simulink model "sampleModel1989"  (R2023a)
settings: Solver=VariableStepAuto  StartTime=0.0  StopTime=10.0  RelTol=1e-3
libraries: hdlsllib x7, simulink x2
settings Model: Creator=user1  LastModifiedBy=user1

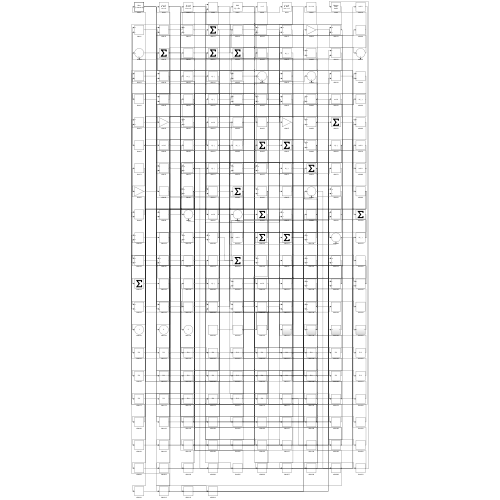
[thumbnail: Simulink's stored preview of the top-level diagram]
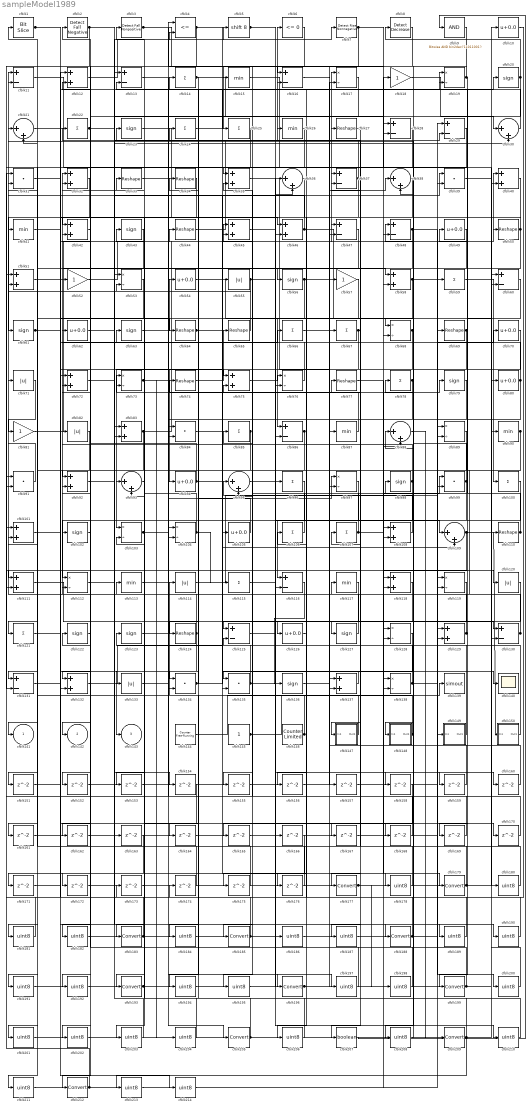
== system sampleModel1989 ==
  cfblk1 : hdlsllib/Logic and Bit Operations/Bit Slice  lidx=7  ridx=0
  cfblk{10,49,54,62,70,80,94,105,126} (9 alike) : Bias  Bias=0.0  SaturateOnIntegerOverflow=off
  cfblk{14,22,24..25,59,66..67,78,85,96,100,106..107,115,121} (15 alike) : Sum  Inputs=+
  cfblk{12,32,35,40,42,45..46,51,58,72,75,83,92,101,108,111,118,129,132,137} (20 alike) : Sum
  cfblk{20,23,43,56,61,63,79,98,102,122..123,127,136} (13 alike) : Signum
  cfblk{17,19,53,68,73,76,89,97,103..104,112,119,128,138} (14 alike) : Product  Inputs=*/  RndMeth=Zero  SaturateOnIntegerOverflow=on
  cfblk{21,30,36,38,88,93,95,109} (8 alike) : Sum  Inputs=|++
  cfblk{11,13,16,28..29,37,47..48,60,86,116,125,130..131} (14 alike) : Sum  Inputs=+-
  cfblk{27,33..34,44,50,64..65,69,74,77,110,124} (12 alike) : Reshape
  cfblk{15,26,41,87,90,113,117} (7 alike) : MinMax
  cfblk{55,71,82,114,120,133} (6 alike) : Abs  SaturateOnIntegerOverflow=off
  cfblk{31,39,84,91,99,134..135} (7 alike) : DotProduct  OutDataTypeStr=Inherit: Inherit via internal rule
  cfblk139 : ToWorkspace  VariableName=simout  SaveFormat=Timeseries  SampleTime=-1
  cfblk140 : Scope
  cfblk144 : hdlsllib/Sources/Counter Free-Running  NumBits=16  tsamp=-1
  cfblk145 : Constant  SampleTime=-1
  cfblk146 : hdlsllib/Sources/Counter Limited  uplimit=7  tsamp=-1
  cfblk147 : Subsystem
      settings: LibrarySourceBlock=|
      | hdlsllib/Ports &
      | Subsystems/Subsystem
  cfblk148 : Subsystem
      settings: LibrarySourceBlock=|
      | hdlsllib/Ports &
      | Subsystems/Subsystem
  cfblk149 : Subsystem
      settings: LibrarySourceBlock=|
      | hdlsllib/Ports &
      | Subsystems/Subsystem
  cfblk150 : Subsystem
      settings: LibrarySourceBlock=|
      | hdlsllib/Ports &
      | Subsystems/Subsystem
  cfblk{151..176} (26 alike) : Delay  SampleTime=1
  cfblk{177,179,183,185,188,193,196,199,205,209,212} (11 alike) : DataTypeConversion  SaturateOnIntegerOverflow=off  RndMeth=Floor
  cfblk{178,180..182,184,186..187,189..192,194..195,197..198,200..204,206,208,210..211,213..214} (26 alike) : DataTypeConversion  OutDataTypeStr=uint8  SaturateOnIntegerOverflow=off  RndMeth=Floor
  cfblk{18,52,57,81} (4 alike) : Gain
  cfblk2 : hdlsllib/Logic and Bit Operations/Detect Fall Negative  vinit=0  OutDataTypeStr=boolean
  cfblk207 : DataTypeConversion  OutDataTypeStr=boolean  SaturateOnIntegerOverflow=off  RndMeth=Floor
  cfblk3 : hdlsllib/Logic and Bit Operations/Detect Fall Nonpositive  vinit=0  OutDataTypeStr=boolean
  cfblk4 : RelationalOperator  Operator=<=  OutDataTypeStr=boolean  InputSameDT=off
  cfblk5 : ArithShift  BitShiftNumber=8
  cfblk6 : hdlsllib/Logic and Bit Operations/Compare To Zero  relop=<=  OutDataTypeStr=boolean
  cfblk7 : hdlsllib/Logic and Bit Operations/Detect Rise Nonnegative  vinit=0  OutDataTypeStr=boolean
  cfblk8 : simulink/Logic and Bit Operations/Detect Decrease  vinit=0.0  OutDataTypeStr=boolean
      settings: LibrarySourceBlock=|
      | hdlsllib/Logic and Bit
      | Operations/Detect
      | Decrease
  cfblk9 : simulink/Logic and Bit Operations/Bitwise Operator  logicop=AND  UseBitMask=on  BitMask=bin2dec('11011001')  BitMaskRealWorld=Stored Integer
      settings: LibrarySourceBlock=|
      | hdlsllib/Logic and Bit
      | Operations/Bitwise
      | Operator
  cfblk141 : Outport  VectorParamsAs1DForOutWhenUnconnected=off
  cfblk142 : Outport  Port=2  VectorParamsAs1DForOutWhenUnconnected=off
  cfblk143 : Outport  Port=3  VectorParamsAs1DForOutWhenUnconnected=off
  wires:
  cfblk46/1 -> cfblk68/1, cfblk11/2
  cfblk79/1 -> cfblk94/1
  cfblk67/1 -> cfblk103/1, cfblk187/1
  cfblk97/1 -> cfblk116/1
  cfblk119/1 -> cfblk185/1
  cfblk81/1 -> cfblk44/1
  cfblk90/1 -> cfblk117/1, cfblk161/1, cfblk201/1
  cfblk91/1 -> cfblk11/1
  cfblk78/1 -> cfblk126/1, cfblk148/1(In1)
  cfblk83/1 -> cfblk17/1, cfblk141/1, cfblk171/1
  cfblk120/1 -> cfblk127/1
  cfblk116/1 -> cfblk136/1
  cfblk38/1 -> cfblk147/1(In1)
  cfblk104/1 -> cfblk32/1, cfblk115/1
  cfblk68/1 -> cfblk93/1, cfblk135/2
  cfblk111/1 -> cfblk129/2
  cfblk7/1 -> cfblk25/1, cfblk83/2, cfblk40/2
  cfblk51/1 -> cfblk58/1
  cfblk52/1 -> cfblk40/1
  cfblk72/1 -> cfblk188/1
  cfblk60/1 -> cfblk199/1
  cfblk63/1 -> cfblk54/1
  cfblk20/1 -> cfblk8/1, cfblk182/1
  cfblk99/1 -> cfblk21/1, cfblk207/1
  cfblk4/1 -> cfblk132/1, cfblk178/1
  cfblk129/1 -> cfblk71/1, cfblk107/1
  cfblk71/1 -> cfblk81/1
  cfblk109/1 -> cfblk150/1(In1), cfblk111/2
  cfblk57/1 -> cfblk86/1
  cfblk31/1 -> cfblk20/1
  cfblk149/1(Out1) -> cfblk98/1
  cfblk80/1 -> cfblk34/1, cfblk167/1
  cfblk32/1 -> cfblk131/1
  cfblk130/1 -> cfblk32/2, cfblk16/2
  cfblk93/1 -> cfblk73/1
  cfblk26/1 -> cfblk131/2
  cfblk24/1 -> cfblk19/1
  cfblk88/1 -> cfblk209/1
  cfblk76/1 -> cfblk62/1
  cfblk61/1 -> cfblk50/1, cfblk64/1
  cfblk11/1 -> cfblk104/1
  cfblk89/1 -> cfblk212/1
  cfblk34/1 -> cfblk61/1
  cfblk82/1 -> cfblk132/2
  cfblk112/1 -> cfblk29/2
  cfblk134/1 -> cfblk14/1, cfblk39/1
  cfblk110/1 -> cfblk49/1, cfblk45/2
  cfblk87/1 -> cfblk33/1
  cfblk125/1 -> cfblk130/1
  cfblk148/1(Out1) -> cfblk114/1, cfblk38/2
  cfblk65/1 -> cfblk23/1
  cfblk59/1 -> cfblk100/1
  cfblk107/1 -> cfblk99/1, cfblk26/1, cfblk120/1
  cfblk56/1 -> cfblk104/2, cfblk38/1
  cfblk48/1 -> cfblk92/1, cfblk200/1
  cfblk96/1 -> cfblk183/1
  cfblk12/1 -> cfblk5/1
  cfblk103/1 -> cfblk7/1, cfblk197/1
  cfblk44/1 -> cfblk6/1
  cfblk58/1 -> cfblk111/1, cfblk190/1
  cfblk75/1 -> cfblk76/1
  cfblk17/1 -> cfblk35/1
  cfblk106/1 -> cfblk85/1
  cfblk145/1 -> cfblk139/1, cfblk97/2
  cfblk77/1 -> cfblk179/1
  cfblk2/1 -> cfblk91/2, cfblk30/2, cfblk28/2
  cfblk30/1 -> cfblk3/1
  cfblk108/1 -> cfblk95/1
  cfblk146/1 -> cfblk101/2, cfblk112/2
  cfblk121/1 -> cfblk52/1
  cfblk94/1 -> cfblk2/1, cfblk109/2
  cfblk98/1 -> cfblk112/1, cfblk82/1
  cfblk144/1 -> cfblk18/1
  cfblk23/1 -> cfblk76/2
  cfblk16/1 -> cfblk87/1
  cfblk84/1 -> cfblk47/1
  cfblk50/1 -> cfblk41/1, cfblk211/1
  cfblk28/1 -> cfblk124/1
  cfblk137/1 -> cfblk135/1
  cfblk74/1 -> cfblk65/1
  cfblk113/1 -> cfblk205/1
  cfblk21/1 -> cfblk80/1
  cfblk8/1 -> cfblk47/2
  cfblk45/1 -> cfblk116/2
  cfblk118/1 -> cfblk125/1
  cfblk25/1 -> cfblk121/1
  cfblk138/1 -> cfblk70/1, cfblk48/1, cfblk75/2
  cfblk35/1 -> cfblk137/2
  cfblk49/1 -> cfblk56/1
  cfblk22/1 -> cfblk4/2, cfblk154/1
  cfblk124/1 -> cfblk143/1, cfblk21/2
  cfblk69/1 -> cfblk19/2, cfblk175/1, cfblk184/1
  cfblk13/1 -> cfblk196/1
  cfblk85/1 -> cfblk142/1, cfblk172/1
  cfblk18/1 -> cfblk30/1
  cfblk114/1 -> cfblk59/1
  cfblk86/1 -> cfblk102/1, cfblk194/1
  cfblk64/1 -> cfblk105/1, cfblk140/1
  cfblk73/1 -> cfblk45/1, cfblk204/1
  cfblk14/1 -> cfblk57/1, cfblk164/1
  cfblk100/1 -> cfblk134/1
  cfblk1/1 -> cfblk46/1, cfblk133/1, cfblk75/1
  cfblk3/1 -> cfblk28/1, cfblk15/1
  cfblk135/1 -> cfblk63/1, cfblk158/1
  cfblk5/1 -> cfblk108/2, cfblk109/1
  cfblk54/1 -> cfblk90/1
  cfblk70/1 -> cfblk84/1
  cfblk150/1(Out1) -> cfblk35/2
  cfblk15/1 -> cfblk67/1
  cfblk147/1(Out1) -> cfblk125/2
  cfblk92/1 -> cfblk37/1
  cfblk131/1 -> cfblk66/1
  cfblk19/1 -> cfblk16/1, cfblk169/1
  cfblk29/1 -> cfblk42/1
  cfblk37/1 -> cfblk22/1, cfblk153/1
  cfblk36/1 -> cfblk193/1
  cfblk127/1 -> cfblk74/1
  cfblk133/1 -> cfblk79/1
  cfblk27/1 -> cfblk177/1
  cfblk55/1 -> cfblk51/2, cfblk210/1
  cfblk123/1 -> cfblk97/1
  cfblk105/1 -> cfblk24/1
  cfblk33/1 -> cfblk84/2
  cfblk132/1 -> cfblk55/1
  cfblk42/1 -> cfblk12/2
  cfblk43/1 -> cfblk151/1
  cfblk151/1 -> cfblk12/1
  cfblk47/1 -> cfblk152/1
  cfblk152/1 -> cfblk108/1
  cfblk153/1 -> cfblk93/2
  cfblk6/1 -> cfblk155/1
  cfblk155/1 -> cfblk46/2
  cfblk126/1 -> cfblk156/1
  cfblk156/1 -> cfblk129/1
  cfblk66/1 -> cfblk157/1
  cfblk157/1 -> cfblk68/2
  cfblk136/1 -> cfblk159/1
  cfblk159/1 -> cfblk137/1
  cfblk115/1 -> cfblk160/1
  cfblk160/1 -> cfblk37/2
  cfblk161/1 -> cfblk99/2
  cfblk122/1 -> cfblk162/1
  cfblk162/1 -> cfblk92/2
  cfblk164/1 -> cfblk48/2
  cfblk128/1 -> cfblk165/1
  cfblk165/1 -> cfblk29/1
  cfblk167/1 -> cfblk58/2
  cfblk101/1 -> cfblk168/1
  cfblk168/1 -> cfblk95/2
  cfblk169/1 -> cfblk51/1
  cfblk62/1 -> cfblk170/1
  cfblk170/1 -> cfblk4/1
  cfblk172/1 -> cfblk138/2
  cfblk173/1 -> cfblk73/2
  cfblk10/1 -> cfblk174/1
  cfblk174/1 -> cfblk1/1
  cfblk175/1 -> cfblk42/2
  cfblk40/1 -> cfblk176/1
  cfblk176/1 -> cfblk103/2
  cfblk177/1 -> cfblk10/1, cfblk198/1
  cfblk178/1 -> cfblk27/1
  cfblk179/1 -> cfblk31/2, cfblk128/1
  cfblk39/1 -> cfblk180/1
  cfblk180/1 -> cfblk77/1
  cfblk166/1 -> cfblk181/1
  cfblk181/1 -> cfblk31/1
  cfblk182/1 -> cfblk166/1
  cfblk183/1 -> cfblk128/2, cfblk91/1
  cfblk184/1 -> cfblk96/1
  cfblk185/1 -> cfblk138/1, cfblk43/1
  cfblk95/1 -> cfblk186/1
  cfblk186/1 -> cfblk119/1
  cfblk187/1 -> cfblk119/2
  cfblk188/1 -> cfblk173/1, cfblk106/1, cfblk83/1
  cfblk171/1 -> cfblk189/1
  cfblk189/1 -> cfblk72/1
  cfblk190/1 -> cfblk72/2
  cfblk163/1 -> cfblk191/1
  cfblk191/1 -> cfblk86/2
  cfblk102/1 -> cfblk192/1
  cfblk192/1 -> cfblk163/1
  cfblk193/1 -> cfblk17/2, cfblk130/2
  cfblk194/1 -> cfblk36/1
  cfblk158/1 -> cfblk195/1
  cfblk195/1 -> cfblk36/2
  cfblk196/1 -> cfblk39/2, cfblk69/1
  cfblk197/1 -> cfblk13/1
  cfblk198/1 -> cfblk13/2
  cfblk199/1 -> cfblk118/1, cfblk122/1
  cfblk200/1 -> cfblk60/1
  cfblk201/1 -> cfblk60/2
  cfblk53/1 -> cfblk202/1
  cfblk202/1 -> cfblk149/1(In1)
  cfblk154/1 -> cfblk203/1
  cfblk203/1 -> cfblk53/1
  cfblk204/1 -> cfblk53/2
  cfblk205/1 -> cfblk110/1, cfblk123/1
  cfblk117/1 -> cfblk206/1
  cfblk206/1 -> cfblk113/1
  cfblk207/1 -> cfblk9/1
  cfblk9/1 -> cfblk208/1
  cfblk208/1 -> cfblk78/1
  cfblk209/1 -> cfblk134/2, cfblk213/1
  cfblk210/1 -> cfblk88/1
  cfblk211/1 -> cfblk88/2
  cfblk212/1 -> cfblk118/2, cfblk101/1
  cfblk213/1 -> cfblk89/1
  cfblk41/1 -> cfblk214/1
  cfblk214/1 -> cfblk89/2

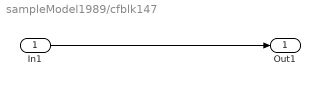
== system sampleModel1989/cfblk147 ==
  In1 : Inport
  Out1 : Outport
  wires:
  In1/1 -> Out1/1

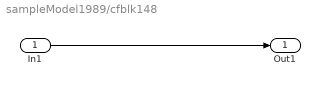
== system sampleModel1989/cfblk148 ==
  In1 : Inport
  Out1 : Outport
  wires:
  In1/1 -> Out1/1

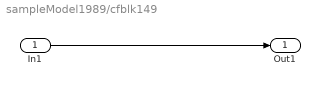
== system sampleModel1989/cfblk149 ==
  In1 : Inport
  Out1 : Outport
  wires:
  In1/1 -> Out1/1

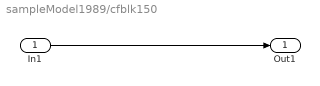
== system sampleModel1989/cfblk150 ==
  In1 : Inport
  Out1 : Outport
  wires:
  In1/1 -> Out1/1
